simulink model "toLightSourceRef"  (R2013b)
settings: Solver=FixedStepDiscrete  StartTime=0.0  StopTime=inf  RelTol=1e-3
libraries: simulink_extras x2
settings Model: Creator=davendano  LastModifiedBy=davendano
settings OptimizationCC: InlineParams=on

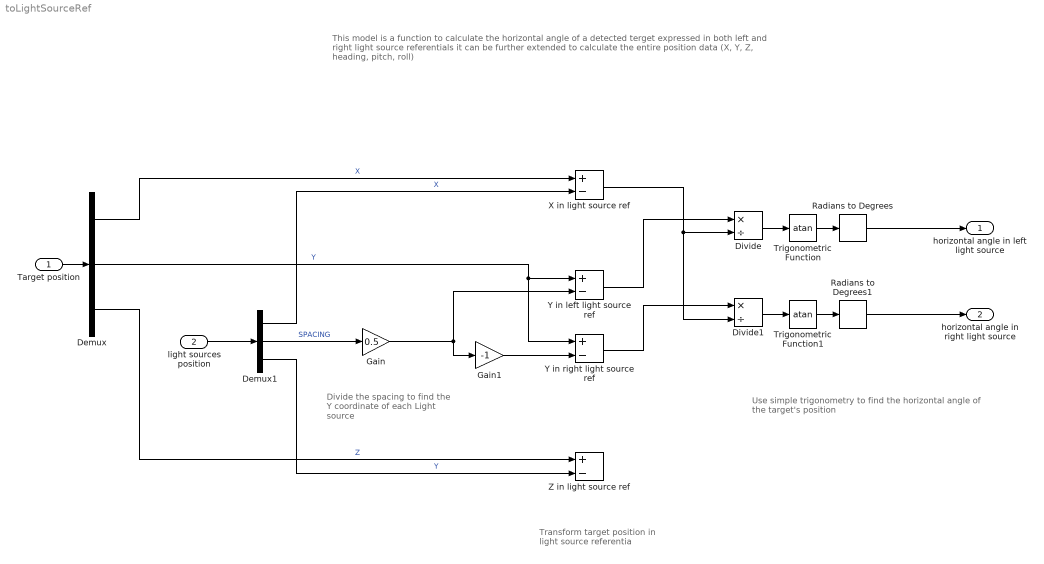
== system toLightSourceRef ==
  note: Divide the spacing to find
      | the Y coordinate of each
      | Light source
  note: Use simple trigonometry to find the horizontal angle
      | of the target's position
  note: Transform target position
      | in light source referentia
  note: This model is a function to calculate the horizontal angle of a detected terget expressed in both left and right light source referentials
      | it can be further extended to calculate the entire position data (X, Y, Z, heading, pitch, roll)
  Target position : Inport
  light sources position : Inport  Port=2
  Demux : Demux  Outputs=3
  Demux1 : Demux  Outputs=3
  Divide : Product  Inputs=*/
  Divide1 : Product  Inputs=*/
  Gain : Gain  Gain=0.5
  Gain1 : Gain  Gain=-1
  Radians to Degrees : simulink_extras/Transformations/Radians to Degrees
  Radians to Degrees1 : simulink_extras/Transformations/Radians to Degrees
  Trigonometric Function : Trigonometry  Operator=atan
  Trigonometric Function1 : Trigonometry  Operator=atan
  X in light source ref : Sum  Inputs=+-
  Y in left light source ref : Sum  Inputs=+-
  Y in right light source ref : Sum  Inputs=+-
  Z in light source ref : Sum  Inputs=+-
  horizontal angle in left light source : Outport
  horizontal angle in right light source : Outport  Port=2
  wires:
  Demux/1 -> X in light source ref/1  "X"
  Demux/2 -> Y in right light source ref/1, Y in left light source ref/1  "Y"
  light sources position/1 -> Demux1/1
  Target position/1 -> Demux/1
  Gain1/1 -> Y in right light source ref/2
  Gain/1 -> Y in left light source ref/2, Gain1/1
  Demux1/2 -> Gain/1  "SPACING"
  Demux1/3 -> Z in light source ref/2  "Y"
  Demux/3 -> Z in light source ref/1  "Z"
  Demux1/1 -> X in light source ref/2  "X"
  Divide/1 -> Trigonometric Function/1
  Trigonometric Function/1 -> Radians to Degrees/1
  Radians to Degrees/1 -> horizontal angle in left light source/1
  Divide1/1 -> Trigonometric Function1/1
  Trigonometric Function1/1 -> Radians to Degrees1/1
  Radians to Degrees1/1 -> horizontal angle in right light source/1
  X in light source ref/1 -> Divide/2, Divide1/2
  Y in right light source ref/1 -> Divide1/1
  Y in left light source ref/1 -> Divide/1
